simulink model "psbmachinesrazdel6"  (Simulink 5.0)
settings: Solver=ode23tb  SolverMode=SingleTasking  StartTime=0.0  StopTime=5  MaxStep=1/60  RelTol=1e-3
undefined symbols (not defined in the file): D1, Delta, st_a, st_b, st_c
libraries: powerlib2 x32, powerlib_extras x1
settings Model: Creator=patrice  LastModifiedBy=pavel  ExtModeTrigMode=oneshot  ExtModeArmWhenConnect=off  ExtModeAutoUpdateStatusClock=off  OutputTimes=[0:1/20:10]  LimitDataPoints=off  BlockReductionOpt=off  BooleanDataType=off  ProdHWWordLengths=8,32,16,32  RTWTemplateMakefile=grt_unix.tmf  RTWOptions="-aEnforceIntegerDowncast=1 -aExtMode=0 -aExtModeTesting=0 -aFoldNonRolledExpr=1 -aForceParamTrailComments=0 -aGenerateComments=1 -aGenerateReport=0 -aIgnoreCustomStorageClasses=0 -aIncDataTypeInIds=0 -aIncHierarchyInIds=0 -aInlineInvariantSignals=0 -aInlinedPrmAccess=\"Literals\" -aLocalBlockOutputs=1 -aLogVarNameModifier=\"rt_\" -aMaxRTWIdLen=31 -aPrefixModelToSubsysFcnNames=1 -aRTWVerbose=1 -aRollThreshold=5 -aShowEliminatedStatements=1"

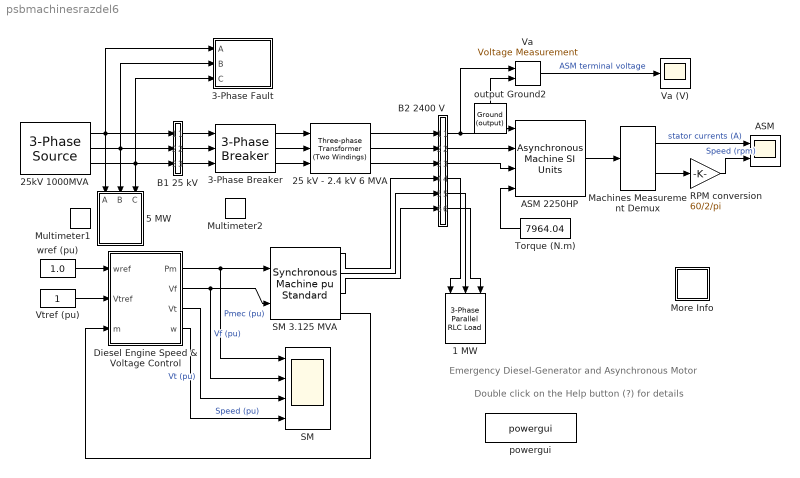
== system psbmachinesrazdel6 ==
  note: Emergency Diesel-Generator and Asynchronous Motor
  note: Double click on the Help button (?) for details
  1 MW : powerlib2/Elements/3-Phase Parallel RLC Load  Orientation=down  Vpp=2400  fn=60  P3=1e6  QL3=0  QC3=0
  25 kV - 2.4 kV 6 MVA : powerlib2/Elements/Three-phase Transformer (Two Windings)  Tag=PoWeRsYsTeMbLoCk  nominal=[ 6e6 , 60 ]  type1=Yg  params1=[ 25e3 , 0.0015 , 0.03]  type2=Delta (D1)  params2=[ 2.4e3 , 0.0015 , 0.03 ]  ynsat=off  rmag=200  lm=200  sat="[ 0,0  ;  0.005,1.2  ;  1.0,1.4 ]"  hyst=off  matfile='hysteresis'  sif=off  phi0=[ 0.8 , -0.8 , 0.7 ]  initialslopes=[+1 +1 +1]  mesure=Winding voltages  PSBOutputType=1111
  25kV 1000MVA : powerlib2/Electrical Sources/3-Phase Source  Tag=PoWeRsYsTeMbLoCk  V=25e3  Phi=0  F=60  InternalConnection=Yg  RLoff=on  R=25^2/1000/10  L=25^2/1000/377  Psc=1000e6  Vbase=25e3  XRratio=10  PSBOutputType=111
  3-Phase Breaker : powerlib2/Elements/3-Phase Breaker  init_states=closed  sa=on  sb=on  sc=on  sw_times=[0.2]  Ts=0  comext=off  Ron=0.01  Rp=1e5  Cp=inf  mesure=Breaker currents
  3-Phase Fault : Subsystem  AncestorBlock=powerlib2/Elements/3-Phase Fault  mask(Three-Phase Fault){sa=on, sb=on, sc=on, Rdef=0.01, st=on, Rt=0.001, comext=off, sw_status=[1 0], sw_times=[ 0.1 0.4], Ts=0, init_statext=[1 1 0], Rp=inf, Cp=inf, mesure=None}
      mask prompts: sa "Phase A Fault"; sb "Phase B Fault"; sc "Phase C Fault"; Rdef "Fault resistances  Ron (ohms) :"; st "Ground Fault"; Rt "Ground resistance Rg (ohms) :"; comext "External control of fault timing :"; sw_status "Transition status [1,0,1 ...):"; sw_times "Transition times (s):"; Ts "Sample time of the internal timer Ts(s):"; init_statext "Initial status of fault [Phase A  Phase B  Phase C]:"; Rp "Snubbers resistance Rp (ohms) :"; Cp "Snubbers Capacitance Cp (Farad)"; mesure "Measurements"
      mask help: Use this block to program a fault (short-circuit) between any phase and the ground. You can define the fault timing directly from the dialog box or apply an external logical signal. If you check the 'External control' box , the external control input will appear.
      mask init:
      | [st_a,st_b,st_c,Rground,init_a,init_b,init_c,p7,p8,p9,p10,p11]=powericon('Three-Phase Fault',Rdef,Rt,sw_times,sw_status,sa,sb,sc,st,init_statext,comext);
      | desc0=setstr(p7);
      | desc1=setstr(p8);
      | desc2=setstr(p9);
      | desc3=setstr(p10);
      | desc4=setstr(p11);
      | powericon('psbcbtransfo',gcb,'Three-phase Fault');
      mask Help: web(psbhelp)
      mask StyleString: checkbox,checkbox,checkbox,edit,checkbox,edit,checkbox,edit,edit,edit,edit,edit,edit,popup(None|Fault voltages|Fault currents|Fault voltages and currents)
      mask CallbackString: ||||powericon('psbcbtransfo',gcb,'Three-phase Fault')||powericon('psbcbtransfo',gcb,'Three-phase Fault')|||||||
      mask Display: disp([desc0,'\n',desc1,desc2,desc3])
  5 MW : Subsystem  Orientation=down  AncestorBlock=powerlib2/Elements/3-Phase Parallel RLC Load  mask(3-phase parallel RLC load ){Vpp=25e3, fn=60, P3=5e6, QL3=0, QC3=0}
      mask prompts: Vpp "Nominal phase-phase voltage (Vrms):"; fn "Nominal frequency (Hz):"; P3 "Three-phase active power P (W):"; QL3 "Three-phase inductive reactive power Ql (var)"; QC3 "Three-phase capacitive reactive power Qc (var) :"
      mask help: This block implements a three-phase parallel RLC load connected in Y configureation, with the neutral connected to the ground. Each phase consist of one parallel RLC load block connected between the phase input and the ground.
      mask init:
      | [p0,p1,p2,p3,p4,p5,p6,p7,p8,p9,p10,p11,p12,p13,p14,p15,p16] = powericon('3-phase parallel RLC load',P3,QL3,QC3);
      mask Help: Look under the mask of the 3-phase parallel RLC load block to see how it is built.
      mask Display: plot(p0-30,p1,p2,p3,p4,p5,p6,p7,p8,p9,p10,p11,p12,p13,p14,p15,[200,200],[-35 35],[215 215],[-25 25],[230 230],[-15 15],[p16,200],[0,0])
  ASM : Scope  NumInputPorts=2
      settings: TimeRange=5  YMin=-3000~-1800  YMax=3000~-1000  DataFormat=Array
  ASM 2250HP : powerlib2/Machines/Asynchronous Machine SI Units  Tag=PoWeRsYsTeMbLoCk  rotType=Squirrel-cage  ctrl=Rotor  x1=[ 2250*746, 2400, 60 ]  x2=[ 0.029 0.226/377]  x3=[ 0.022 0.226/377]  x4=13.04/377  x5="[ 63.87 0  2 ]"  x6=[0.00611928 0 556.114 556.114 556.114 -53.6639 -173.664 66.3361]  PSBOutputType=1110  iounits=1  LoadFlowParameters=1492000
  B1 25 kV : Subsystem
      mask Display: disp('')
  B2 2400 V : Subsystem
      mask Display: disp('')
  Diesel Engine Speed & Voltage Control : Subsystem
  Machines Measurement Demux : powerlib2/Machines/Machines Measurement Demux  machType=Asynchronous  ssm1=on  ssm2=on  ssm3=on  ssm4=on  ssm5=on  ssm6=on  sm1=on  sm2=on  sm3=on  sm4=on  sm5=on  sm6=on  sm7=on  sm8=on  sm9=on  sm10=on  sm11=on  sm115=off  sm12=off  sm13=off  sm14=off  asm1=off  asm2=off  asm3=off  asm4=off  asm5=on  asm6=off  asm7=off  asm8=off  asm9=on  asm10=off  asm11=off  pmsm1=on  pmsm2=on  pmsm3=on  pmsm4=on  pmsm5=on  pmsm6=on  lastType=1
  More Info : Subsystem
      mask Display: disp('?')
  Multimeter1 : powerlib2/Measurements/Multimeter  Tag=PoWeRsYsTeMmEaSuReMeNt  PhasorSimulation=off  OutputType=Magnitude  sel=[7 8 9]  L=12  Gain=[1 1 1]  yselected={'Ib: 5 MW/Parallel RLC Load 1','Ib: 5 MW/Parallel RLC Load 2','Ib: 5 MW/Parallel RLC Load 3'};  PSBOutputType=1  PSBequivalent=0  AxesSetting=[0,0.1,-100,100]  Display=0  SavedBlockNames=-11
  Multimeter2 : powerlib2/Measurements/Multimeter  Tag=PoWeRsYsTeMmEaSuReMeNt  PhasorSimulation=off  OutputType=Magnitude  sel=[10 11 12]  L=12  Gain=[1 1 1]  yselected={'Ib: 3-Phase Breaker/Breaker A','Ib: 3-Phase Breaker/Breaker B','Ib: 3-Phase Breaker/Breaker C'};  PSBOutputType=1  PSBequivalent=0  AxesSetting=[0,0.1,-100,100]  Display=0  SavedBlockNames=-11
  RPM conversion : Gain  Gain=60/2/pi  SaturateOnIntegerOverflow=on
  SM : Scope  NumInputPorts=4
      settings: YMin=0~0~0~0  YMax=1.5~6~1.5~1.2  SaveName=Pmec_SM  DataFormat=Structure  Decimation=10
  SM 3.125 MVA : powerlib2/Machines/Synchronous Machine pu Standard  Tag=PoWeRsYsTeMbLoCk  rotorType=Salient-pole  x1="[ 3.125e6  2400  60 ]"  x2b=[ 31 32 33 34 35 36 37 ]  x2=[ 1.56, 0.296, 0.177, 1.06, 0.177, 0.052 ]  dAxisT=Short-circuit  qAxisT=Open-circuit  x3a=[]  x3b=[]  x3c=[]  x3d=[]  x3=[ 3.7, 0.05, 0.05 ]  x3e=[]  x3f=[]  x3g=[]  x4=0.0036  x5="[ 1.07  0  2 ]"  x6=[0 -114.05 0.306018 0.306018 0.306018 -90.0504 149.95 29.9496 1.42796]  x7=off  x8=[0.211 0.418 1.0 1.72 3.35 ; 0.25 0.50 1.0 1.2 1.4]  PSBOutputType=1110  iounits=0.5  LoadFlowParameters=[1 500000 0 0]
  Torque (N.m) : Constant  Orientation=left  Value=7964.04
  Va : powerlib2/Measurements/Voltage Measurement  Tag=PoWeRsYsTeMmEaSuReMeNt  PhasorSimulation=off  OutputType=Magnitude  PSBOutputType=0  PSBequivalent=1
  Va (V) : Scope
      settings: TickLabels=on  TimeRange=0.2  YMin=-2000  YMax=2000  DataFormat=Array
  Vtref (pu) : Constant
  output Ground2 : powerlib2/Connectors/Ground (output)  Tag=PoWeRsYsTeMbLoCk  Orientation=up  PSBOutputType=1
  powergui : powerlib2/powergui  Frange=logspace(0,3,50)  Ylog=off  Xlog=off  save=off  variable=ZData  ZoomFFT=on  StartTime=0.0  cycles=2  DisplayStyle=off  fundamental=60  FreqAxis=off  MaxFrequency=1000  frequencyindice=60  frequencyindicesteady=1  RmsSteady=1  display=off  Ts=0  methode=off  frequency=60  echomessages=off
  wref (pu) : Constant  Value=1.0
  wires:
  25kV 1000MVA/3 -> 3-Phase Fault/3(C), 5 MW/3(C), B1 25 kV/3(C1)
  25kV 1000MVA/2 -> 3-Phase Fault/2(B), 5 MW/2(B), B1 25 kV/2(B1)
  25kV 1000MVA/1 -> 3-Phase Fault/1(A), 5 MW/1(A), B1 25 kV/1(A1)
  B1 25 kV/3(C2) -> 3-Phase Breaker/3
  B1 25 kV/2(B2) -> 3-Phase Breaker/2
  B1 25 kV/1(A2) -> 3-Phase Breaker/1
  3-Phase Breaker/1 -> 25 kV - 2.4 kV 6 MVA/1
  wref (pu)/1 -> Diesel Engine Speed & Voltage Control/1(wref)
  SM 3.125 MVA/4 -> Diesel Engine Speed & Voltage Control/3(m)
  Vtref (pu)/1 -> Diesel Engine Speed & Voltage Control/2(Vtref)
  3-Phase Breaker/3 -> 25 kV - 2.4 kV 6 MVA/3
  3-Phase Breaker/2 -> 25 kV - 2.4 kV 6 MVA/2
  25 kV - 2.4 kV 6 MVA/3 -> B2 2400 V/3(C1)
  25 kV - 2.4 kV 6 MVA/2 -> B2 2400 V/2(B1)
  25 kV - 2.4 kV 6 MVA/1 -> B2 2400 V/1(A1`)
  SM 3.125 MVA/1 -> B2 2400 V/4(A2)
  SM 3.125 MVA/2 -> B2 2400 V/5(B2)
  SM 3.125 MVA/3 -> B2 2400 V/6(C2)
  B2 2400 V/1(A3) -> Va/1, ASM 2250HP/1
  Torque (N.m)/1 -> ASM 2250HP/4
  ASM 2250HP/1 -> Machines Measurement Demux/1
  B2 2400 V/5(B4) -> 1 MW/2
  B2 2400 V/2(B3) -> ASM 2250HP/2
  B2 2400 V/3(C3) -> ASM 2250HP/3
  Va/1 -> Va (V)/1  "ASM terminal voltage"
  output Ground2/1 -> Va/2
  Diesel Engine Speed & Voltage Control/1(Pm) -> SM 3.125 MVA/1, SM/1  "Pmec (pu)"
  Diesel Engine Speed & Voltage Control/2(Vf) -> SM 3.125 MVA/2, SM/2  "Vf (pu)"
  Diesel Engine Speed & Voltage Control/3(Vt) -> SM/3  "Vt (pu)"
  Diesel Engine Speed & Voltage Control/4(w) -> SM/4  "Speed (pu)"
  Machines Measurement Demux/2 -> RPM conversion/1
  Machines Measurement Demux/1 -> ASM/1  "stator currents (A)"
  RPM conversion/1 -> ASM/2  "Speed (rpm)"
  B2 2400 V/6(C4) -> 1 MW/3
  B2 2400 V/4(A4) -> 1 MW/1

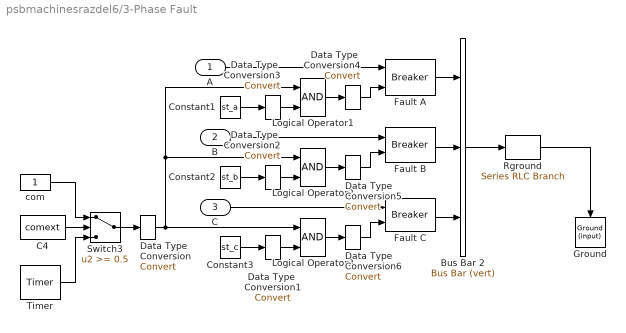
== system psbmachinesrazdel6/3-Phase Fault ==
  A : Inport
  B : Inport  Port=2
  C : Inport  Port=3
  Bus Bar 2 : powerlib2/Connectors/Bus Bar (vert)  Tag=PoWeRsYsTeMbLoCk  entrees=3  sorties=1  PSBOutputType=11111111111111111111111111111111111111111111111111111111111111111111111111111111111111111
  C4 : Constant  Value=comext
  Constant1 : Constant  Value=st_a
  Constant2 : Constant  Value=st_b
  Constant3 : Constant  Value=st_c
  Data Type  Conversion{,1..3} (4 alike) : DataTypeConversion  DataType=boolean  SaturateOnIntegerOverflow=on
  Data Type  Conversion4 : DataTypeConversion  DataType=double  SaturateOnIntegerOverflow=on
  Data Type  Conversion5 : DataTypeConversion  DataType=double  SaturateOnIntegerOverflow=on
  Data Type  Conversion6 : DataTypeConversion  DataType=double  SaturateOnIntegerOverflow=on
  Fault A : powerlib2/Elements/Breaker  Tag=PoWeRsYsTeMbLoCk  a=Rdef  c=init_a  rs=Rp  cs=Cp  times="[ 4/60  5/60 ]"  Ts=0  comext=on  mesure=None  PSBOutputType=1
  Fault B : powerlib2/Elements/Breaker  Tag=PoWeRsYsTeMbLoCk  a=Rdef  c=init_b  rs=Rp  cs=Cp  times="[ 4/60  5/60 ]"  Ts=0  comext=on  mesure=None  PSBOutputType=1
  Fault C : powerlib2/Elements/Breaker  Tag=PoWeRsYsTeMbLoCk  a=Rdef  c=init_c  rs=Rp  cs=Cp  times="[ 4/60  5/60 ]"  Ts=0  comext=on  mesure=None  PSBOutputType=1
  Ground : powerlib2/Connectors/Ground (input)  Tag=PoWeRsYsTeMbLoCk  Orientation=down
  Logical Operator1 : Logic
  Logical Operator2 : Logic
  Logical Operator3 : Logic
  Rground : powerlib2/Elements/Series RLC Branch  Tag=PoWeRsYsTeMbLoCk  a=Rground  b=0  c=inf  mesure=None  PSBOutputType=1
  Switch3 : Switch  Threshold=0.5  InputSameDT=on
  Timer : powerlib_extras/Control  Blocks/Timer  t=sw_times  e=sw_status
  com : Constant
  wires:
  com/1 -> Switch3/1
  Timer/1 -> Switch3/3
  C4/1 -> Switch3/2
  Fault A/1 -> Bus Bar 2/1
  A/1 -> Fault A/1
  Fault C/1 -> Bus Bar 2/3
  Fault B/1 -> Bus Bar 2/2
  B/1 -> Fault B/1
  C/1 -> Fault C/1
  Rground/1 -> Ground/1
  Bus Bar 2/1 -> Rground/1
  Switch3/1 -> Data Type  Conversion/1
  Data Type  Conversion/1 -> Logical Operator3/1, Logical Operator2/1, Logical Operator1/1
  Constant3/1 -> Data Type  Conversion1/1
  Data Type  Conversion1/1 -> Logical Operator3/2
  Constant2/1 -> Data Type  Conversion2/1
  Data Type  Conversion2/1 -> Logical Operator2/2
  Constant1/1 -> Data Type  Conversion3/1
  Data Type  Conversion3/1 -> Logical Operator1/2
  Logical Operator1/1 -> Data Type  Conversion4/1
  Data Type  Conversion4/1 -> Fault A/2
  Logical Operator2/1 -> Data Type  Conversion5/1
  Data Type  Conversion5/1 -> Fault B/2
  Logical Operator3/1 -> Data Type  Conversion6/1
  Data Type  Conversion6/1 -> Fault C/2

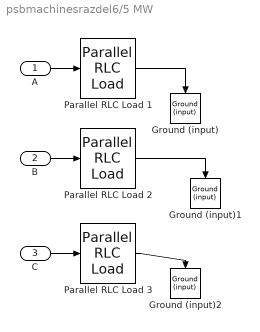
== system psbmachinesrazdel6/5 MW ==
  A : Inport
  B : Inport  Port=2
  C : Inport  Port=3
  Ground (input) : powerlib2/Connectors/Ground (input)  Tag=PoWeRsYsTeMbLoCk  Orientation=down
  Ground (input)1 : powerlib2/Connectors/Ground (input)  Tag=PoWeRsYsTeMbLoCk  Orientation=down
  Ground (input)2 : powerlib2/Connectors/Ground (input)  Tag=PoWeRsYsTeMbLoCk  Orientation=down
  Parallel RLC Load 1 : powerlib2/Elements/Parallel RLC Load  Tag=PoWeRsYsTeMbLoCk  a=Vpp/sqrt(3)  b=fn  c=P3/3  d=QL3/3  e=QC3/3  mesure=Branch current  PSBOutputType=1
  Parallel RLC Load 2 : powerlib2/Elements/Parallel RLC Load  Tag=PoWeRsYsTeMbLoCk  a=Vpp/sqrt(3)  b=fn  c=P3/3  d=QL3/3  e=QC3/3  mesure=Branch current  PSBOutputType=1
  Parallel RLC Load 3 : powerlib2/Elements/Parallel RLC Load  Tag=PoWeRsYsTeMbLoCk  a=Vpp/sqrt(3)  b=fn  c=P3/3  d=QL3/3  e=QC3/3  mesure=Branch current  PSBOutputType=1
  wires:
  C/1 -> Parallel RLC Load 3/1
  Parallel RLC Load 3/1 -> Ground (input)2/1
  B/1 -> Parallel RLC Load 2/1
  Parallel RLC Load 2/1 -> Ground (input)1/1
  A/1 -> Parallel RLC Load 1/1
  Parallel RLC Load 1/1 -> Ground (input)/1

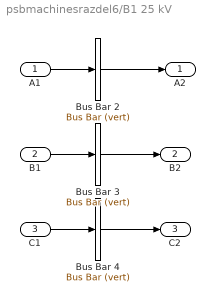
== system psbmachinesrazdel6/B1 25 kV ==
  A1 : Inport
  B1 : Inport  Port=2
  C1 : Inport  Port=3
  Bus Bar 2 : powerlib2/Connectors/Bus Bar (vert)  Tag=PoWeRsYsTeMbLoCk  entrees=1  sorties=1  PSBOutputType=11111111111111111111111111111111111111111111111111111111111111111111111111111111111111111
  Bus Bar 3 : powerlib2/Connectors/Bus Bar (vert)  Tag=PoWeRsYsTeMbLoCk  entrees=1  sorties=1  PSBOutputType=11111111111111111111111111111111111111111111111111111111111111111111111111111111111111111
  Bus Bar 4 : powerlib2/Connectors/Bus Bar (vert)  Tag=PoWeRsYsTeMbLoCk  entrees=1  sorties=1  PSBOutputType=11111111111111111111111111111111111111111111111111111111111111111111111111111111111111111
  A2 : Outport  InitialOutput=0
  B2 : Outport  Port=2  InitialOutput=0
  C2 : Outport  Port=3  InitialOutput=0
  wires:
  Bus Bar 4/1 -> C2/1
  C1/1 -> Bus Bar 4/1
  Bus Bar 3/1 -> B2/1
  B1/1 -> Bus Bar 3/1
  Bus Bar 2/1 -> A2/1
  A1/1 -> Bus Bar 2/1

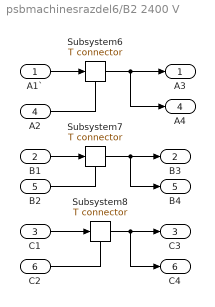
== system psbmachinesrazdel6/B2 2400 V ==
  A1` : Inport
  B1 : Inport  Port=2
  C1 : Inport  Port=3
  A2 : Inport  Port=4
  B2 : Inport  Port=5
  C2 : Inport  Port=6
  Subsystem6 : powerlib2/Connectors/T connector  Tag=PoWeRsYsTeMbLoCk  PSBOutputType=1
  Subsystem7 : powerlib2/Connectors/T connector  Tag=PoWeRsYsTeMbLoCk  PSBOutputType=1
  Subsystem8 : powerlib2/Connectors/T connector  Tag=PoWeRsYsTeMbLoCk  PSBOutputType=1
  A3 : Outport  InitialOutput=0
  B3 : Outport  Port=2  InitialOutput=0
  C3 : Outport  Port=3  InitialOutput=0
  A4 : Outport  Port=4  InitialOutput=0
  B4 : Outport  Port=5  InitialOutput=0
  C4 : Outport  Port=6  InitialOutput=0
  wires:
  A1`/1 -> Subsystem6/1
  C1/1 -> Subsystem8/1
  B1/1 -> Subsystem7/1
  B2/1 -> Subsystem7/Enable
  A2/1 -> Subsystem6/Enable
  C2/1 -> Subsystem8/Enable
  Subsystem6/1 -> A3/1, A4/1
  Subsystem7/1 -> B3/1, B4/1
  Subsystem8/1 -> C3/1, C4/1

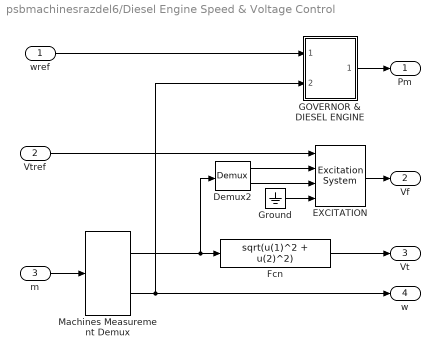
== system psbmachinesrazdel6/Diesel Engine Speed & Voltage Control ==
  wref : Inport
  Vtref : Inport  Port=2
  m : Inport  Port=3
  Demux2 : Demux  Outputs=2
  EXCITATION : powerlib2/Machines/Excitation System  tr=20e-3  reg=[ 200, 0.02 ]  exc=[ 1, 0 ]  tgr=[ 0, 0 ]  damp=[ 0.001, 0.1 ]  sat=[ 0, 0 ]  lim=[ 0, 6, 0 ]  v0=[1,1.182 ]
  Fcn : Fcn  Expr=sqrt(u(1)^2 + u(2)^2)
  GOVERNOR & DIESEL ENGINE : Subsystem  mask(Diesel Engine & Governor){K=40, Tr=[0.01 0.02 0.2], Ta=[0.25 0.009 0.0384], Tlim=[0 1.1], Td=0.024, Pm0=0.160337}
      mask prompts: K "Regulator gain K:"; Tr "Regulator time constants [T1 T2 T3 ] (s) :"; Ta "Actuator time constants [T4 T5 T6] (s) :"; Tlim "Torque limits [Tmin Tmax] (pu) :"; Td "Engine time delay Td (s) :"; Pm0 "Initial value of mechanical power  Pm0 (pu) :"
      mask help:
      | This block implements a diesel engine and governor system:
      | 1st and 2nd inputs: Desired and actual speed (pu)
      | Output: Diesel engine mechanical power.Motor inertia should be combined with generator.
      | Controller transfer function:
      |      Hc=K.(1+T3.s)/(1+T1.s+T1.T2.s^2)
      | Actuator transfer function :
      |      Ha= (1+T4.s) / [ (s (1+T5.s)(1+T6.s) ]
      | Motor :
      |      Time delay Td
      |
      | (See reference in Tutorial Session 5)
  Ground : Ground
  Machines Measurement Demux : powerlib2/Machines/Machines Measurement Demux  machType=Synchronous  ssm1=on  ssm2=on  ssm3=on  ssm4=on  ssm5=on  ssm6=on  sm1=off  sm2=off  sm3=off  sm4=off  sm5=off  sm6=on  sm7=off  sm8=on  sm9=off  sm10=off  sm11=off  sm115=off  sm12=off  sm13=off  sm14=off  asm1=off  asm2=off  asm3=off  asm4=off  asm5=on  asm6=off  asm7=off  asm8=off  asm9=on  asm10=off  asm11=off  pmsm1=on  pmsm2=on  pmsm3=on  pmsm4=on  pmsm5=on  pmsm6=on  lastType=1
  Pm : Outport  InitialOutput=0
  Vf : Outport  Port=2  InitialOutput=0
  Vt : Outport  Port=3  InitialOutput=0
  w : Outport  Port=4  InitialOutput=0
  wires:
  Ground/1 -> EXCITATION/4
  m/1 -> Machines Measurement Demux/1
  Machines Measurement Demux/2 -> GOVERNOR & DIESEL ENGINE/2(w (pu)), w/1
  wref/1 -> GOVERNOR & DIESEL ENGINE/1(wref (pu))
  Demux2/2 -> EXCITATION/3
  EXCITATION/1 -> Vf/1
  GOVERNOR & DIESEL ENGINE/1(Pmec (pu)) -> Pm/1
  Vtref/1 -> EXCITATION/1
  Demux2/1 -> EXCITATION/2
  Machines Measurement Demux/1 -> Demux2/1, Fcn/1
  Fcn/1 -> Vt/1

== system psbmachinesrazdel6/More Info ==
  note: Open the SM and ASM scopes displaying the synchronous machine and asynchronous machine signals.  Start the simulation.
      | Observe that during the fault the terminal voltage drops to about 0.2 pu and the excitation voltage hits the limit of 6 pu. After fault clearing and islanding
      | the SM  mechanical power  increases from its initial value of  0 pu to the final value of 0.80 pu required by the resistive and motor load (2.49 MW) . After 3 seconds,
      | the terminal voltage stabilizes at 1 pu. The motor speed decreases transiently from 1789 rpm to 1635 rpm, then it recovers close to its normal value after 2 seconds.
      |
      | If you  increase the fault duration to 12 cycles by changing the breaker opening time to 0.3 s, you will notice that the system collapses.
      | The ASM speed slows down to zero after 2 seconds.
  note: 3
  note: 1
  note: Demonstration
  note: Circuit Description
  note: This demonstration illustrates fault and islanding of an induction motor/diesel-generator system
      | and demonstrates the Machine Load Flow option of the Powergui.  (See Tutorial Session 7)
  note: A plant consisting of a resistive and motor load (ASM) is fed at 2400 V from a distibution 25 kV network through a 6 MVA 25/2 kV Wye-Delta transformer and from an
      | emergency synchronous generator/ diesel engine unit (SM). The 25 kV network is modelled by a simple R-L equivalent source (short-circuit level 1000 MVA) and a 5 MW load.
      | The  asynchronous motor is  rated 2250 HP, 2.4 kV and the synchronous machine is rated 3.125 MVA, 2.4kV. The SM excitation is performed by the standard
      | excitation block provided in the machine library. The diesel engine and governor system are modelled by a Simulink block (See tutorial, session 7 in the User`s Guide).
      | Initially, the motor develops a mechanical power of 2000 HP (1.49 MW) and the diesel generator is in standby, providing no active power.The synchronous machine excitation
      | system controls the 2400 V bus B2 voltage at 1 pu .  At t = 0.1 s, a three-phase to ground fault occurs on the 25 kV system, causing opening of the 25kV circuit breaker at t = 0.2 s.
      |
      | The demonstration illustrates the mechanical and electrical transients following the fault and islanding of the Motor/Generator system.
  note: Start Simulation. If the SM and ASM initial conditions are not properly set you  will  observe that the voltage and currents Machine do not start in steady state.
      | Stop the simulation.
  note: 2
  note: In order to start the simulation in steady-state you must initialize the synchronous machine and the asynchronous motor for the desired load flow.
      | Open the  Powergui and select "Load Flow & Machine initialization" . The machine "Bus type" should be already initialized as "PV generator",
      | indicating that  the load flow will be performed with the machine controlling its active power and terminal voltage. Specify the desired values by entering
      | the following parameters:
  note: The diesel engine governor and SM excitation system contain integrators and transfer functions which have also been initialized  by the load flow.
      | Open the GOVERNOR block in the Diesel Engine subsystem. Note that the initial mechanical power has been automatically set to 0.00027 pu (844 W).
      | Now open the EXCITATION block. Notice in the last line of the block menu that the initial terminal voltage Vt0 and field voltage Vf0  have been set respectively to
      | 1.0 and 1.4273 pu.The value of the constant block connnected to the  torque input of the asynchronous motor has also been automatically set to 7964 N.
  note: 4
  note: G. Sybille (Hydro-Québec)
  note: Load Flow : U AB (Vrms) = 2400 P (wattts) = 0. Specify also the ASM mechanical power by entering Pmec (Watts) = 2000*746.
  note: Then press the "Execute Load Flow" button.
      |
      | Once the load flow is solved the three line-to-line machine voltages and the three machine currents are updated.
      | The SM reactive power,  mechanical power and  field voltage are displayed : Q = 856 kvar; Pmec = 844 W (power required by resistive losses in stator winding ) ;
      |  field voltage Ef = 1.4273 pu; The active and reactive powers absorbed by the motor, slip and torque are also displayed.

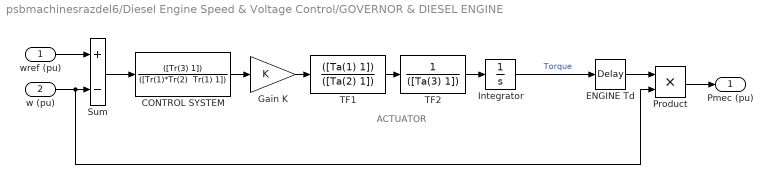
== system psbmachinesrazdel6/Diesel Engine Speed & Voltage Control/GOVERNOR & DIESEL ENGINE ==
  note: ACTUATOR
  wref (pu) : Inport
  w (pu) : Inport  Port=2
  CONTROL SYSTEM : TransferFcn  Numerator=([Tr(3) 1])  Denominator="([Tr(1)*Tr(2)  Tr(1) 1])"
  ENGINE Td : TransportDelay  DelayTime=Td  InitialInput=Pm0
  Gain K : Gain  Gain=K  SaturateOnIntegerOverflow=on
  Integrator : Integrator  InitialCondition=Pm0  LimitOutput=on  UpperSaturationLimit=Tlim(2)  LowerSaturationLimit=Tlim(1)
  Product : Product  SaturateOnIntegerOverflow=on  InputSameDT=on
  Sum : Sum  Inputs=+-  SaturateOnIntegerOverflow=on  InputSameDT=on
  TF1 : TransferFcn  Numerator=([Ta(1) 1])  Denominator=([Ta(2) 1])
  TF2 : TransferFcn  Numerator=1  Denominator=([Ta(3) 1])
  Pmec (pu) : Outport  InitialOutput=0
  wires:
  Gain K/1 -> TF1/1
  Sum/1 -> CONTROL SYSTEM/1
  CONTROL SYSTEM/1 -> Gain K/1
  TF1/1 -> TF2/1
  w (pu)/1 -> Product/2, Sum/2
  ENGINE Td/1 -> Product/1
  wref (pu)/1 -> Sum/1
  Product/1 -> Pmec (pu)/1
  TF2/1 -> Integrator/1
  Integrator/1 -> ENGINE Td/1  "Torque"
